simulink model "dialysisDemo"  (R2023a)
settings: Solver=VariableStepAuto  StartTime=0.0  StopTime=3600*4  RelTol=1e-3
libraries: SignalEditorBlockLib x3
settings Model: PacingRate=500  Creator=alibacon  LastModifiedBy=ppatel
settings DebuggingCC: SubsystemReferenceDiagnosticForUnitTest=warning

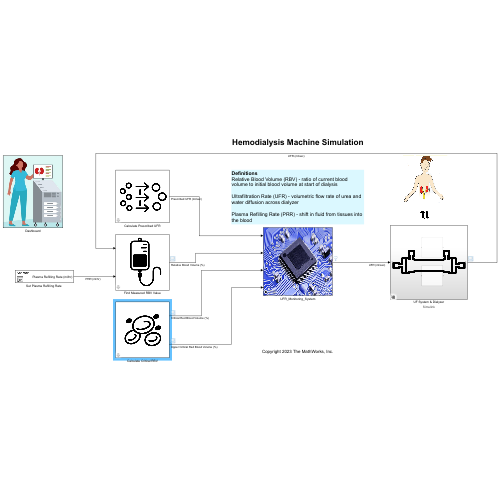
[thumbnail: Simulink's stored preview of the top-level diagram]
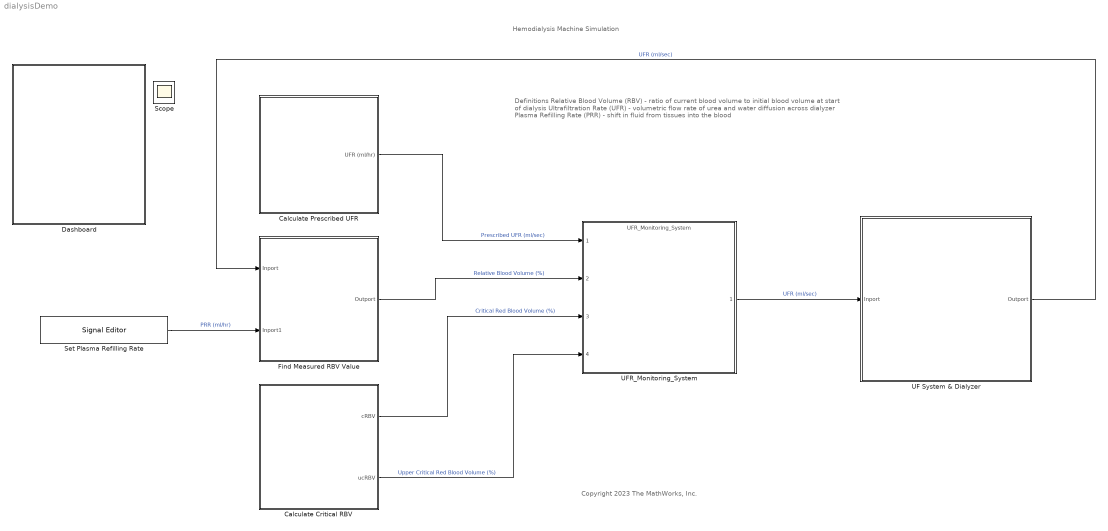
== system dialysisDemo ==
  note: Hemodialysis Machine Simulation
  note: Copyright 2023 The MathWorks, Inc.
  note: Definitions
      | Relative Blood Volume (RBV) - ratio of current blood volume to initial blood volume at start of dialysis
      |
      | Ultrafiltration Rate (UFR) - volumetric flow rate of urea and water diffusion across dialyzer
      |
      | Plasma Refilling Rate (PRR) - shift in fluid from tissues into the blood
  Calculate Critical RBV : Subsystem  mask{BPd=80, UF=2.6, DW=70.6, age=69, arrh=0, chf=0}
      mask prompts: BPd "Diastolic Blood Pressure (mmHg)"; UF "Target Ultrafiltration Volume (L)"; DW "Target Post-Dialysis Dry Weight (kg)"; age "Age (years)"; arrh "Prevalance of Arrythmia"; chf "Prevalance of Congestive Heart Failure Diagnosis"
      mask Display: image('medical-icons-red-blood-cell.png'); % Use "Edit Image" on toolstrip to change.
  Calculate Prescribed UFR : Subsystem  mask{predw=73.2, postdw=70.6, dtime=4}
      mask prompts: predw "Pre-Dialysis Weight (kg)"; postdw "Post-Dialysis Weight (kg)"; dtime "Dialysis Treatment Time (hr)"
      mask Display: image('medical-icons-ufr.png'); % Use "Edit Image" on toolstrip to change.
  Dashboard : Subsystem
      mask Display: image('Dashboard_Input.jpg'); % Use "Edit Image" on toolstrip to change.
  Find Measured RBV Value : Subsystem  mask{BV0=3.774}
      mask prompts: BV0 "Initial Blood Volume (L)"
      mask Display: image('medical-icons-iv-bag.png'); % Use "Edit Image" on toolstrip to change.
  "Set Plasma Refilling Rate " : SignalEditorBlockLib/Signal Editor  FileName=dialysisDemo_PRR.mat  ActiveScenario=Scenario  ActiveSignal=Plasma Refilling Rate (ml/hr)  IsBus=off  OutputBusObjectStr=Bus: BusObject  SampleTime=0  Interpolate=off  ZeroCross=off  OutputAfterFinalValue=Setting to zero  Unit=inherit  PreserveSignalName=on  ApplySigPropsToAllScenarios=on
  UF System & Dialyzer : Subsystem  Variant=on  VariantControlMode=label  VariantControl=Choice  LabelModeActiveChoice=Simulink
      settings: AttributesFormatString=%<LabelModeActiveChoice>
  UFR_Monitoring_System : ModelReference  ModelNameDialog=UFR_Monitoring_System  SimulationMode=Normal  ModelReferenceVersion=3.74
      mask Display: image('Microcontroller.webp'); % Use "Edit Image" on toolstrip to change.
  Scope : Scope
  wires:
  "Set Plasma Refilling Rate "/1 -> Find Measured RBV Value/2(Inport1)  "PRR (ml/hr)"
  UFR_Monitoring_System/1 -> UF System & Dialyzer/1(Inport)  "UFR (ml/sec)"
  UF System & Dialyzer/1(Outport) -> Find Measured RBV Value/1(Inport)  "UFR (ml/sec)"
  Calculate Prescribed UFR/1(UFR (ml/hr)) -> UFR_Monitoring_System/1  "Prescribed UFR (ml/sec)"
  Find Measured RBV Value/1(Outport) -> UFR_Monitoring_System/2  "Relative Blood Volume (%)"
  Calculate Critical RBV/1(cRBV) -> UFR_Monitoring_System/3  "Critical Red Blood Volume (%)"
  Calculate Critical RBV/2(ucRBV) -> UFR_Monitoring_System/4  "Upper Critical Red Blood Volume (%)"

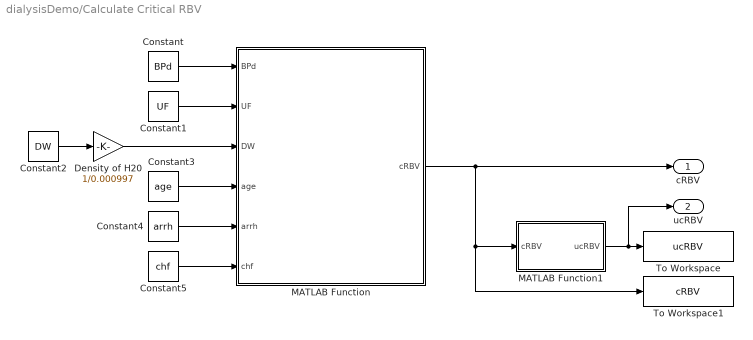
== system dialysisDemo/Calculate Critical RBV ==
  Constant : Constant  Value=BPd
  Constant1 : Constant  Value=UF
  Constant2 : Constant  Value=DW
  Constant3 : Constant  Value=age
  Constant4 : Constant  Value=arrh
  Constant5 : Constant  Value=chf
  Density of H20 : Gain  Gain=1/0.000997
  MATLAB Function : MATLAB Function  TreatAsAtomicUnit=on
  MATLAB Function1 : MATLAB Function  TreatAsAtomicUnit=on
  To Workspace : ToWorkspace  VariableName=ucRBV  SampleTime=-1
  To Workspace1 : ToWorkspace  VariableName=cRBV  SampleTime=-1
  cRBV : Outport
  ucRBV : Outport  Port=2
  wires:
  Constant/1 -> MATLAB Function/1(BPd)
  Constant5/1 -> MATLAB Function/6(chf)
  Constant4/1 -> MATLAB Function/5(arrh)
  Constant3/1 -> MATLAB Function/4(age)
  Constant2/1 -> Density of H20/1
  Constant1/1 -> MATLAB Function/2(UF)
  Density of H20/1 -> MATLAB Function/3(DW)
  MATLAB Function1/1(ucRBV) -> ucRBV/1, To Workspace/1
  MATLAB Function/1(cRBV) -> cRBV/1, To Workspace1/1, MATLAB Function1/1(cRBV)

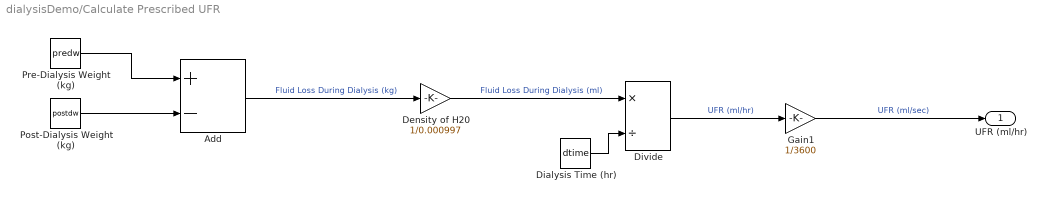
== system dialysisDemo/Calculate Prescribed UFR ==
  Add : Sum  Inputs=+-
  Density of H20 : Gain  Gain=1/0.000997
  Dialysis Time (hr) : Constant  Value=dtime
  Divide : Product  Inputs=*/
  Gain1 : Gain  Gain=1/3600
  Post-Dialysis Weight (kg) : Constant  Value=postdw
  Pre-Dialysis Weight (kg) : Constant  Value=predw
  UFR (ml/hr) : Outport
  wires:
  Add/1 -> Density of H20/1  "Fluid Loss During Dialysis (kg)"
  Divide/1 -> Gain1/1  "UFR (ml/hr)"
  Pre-Dialysis Weight (kg)/1 -> Add/1
  Density of H20/1 -> Divide/1  "Fluid Loss During Dialysis (ml)"
  Post-Dialysis Weight (kg)/1 -> Add/2
  Dialysis Time (hr)/1 -> Divide/2
  Gain1/1 -> UFR (ml/hr)/1  "UFR (ml/sec)"

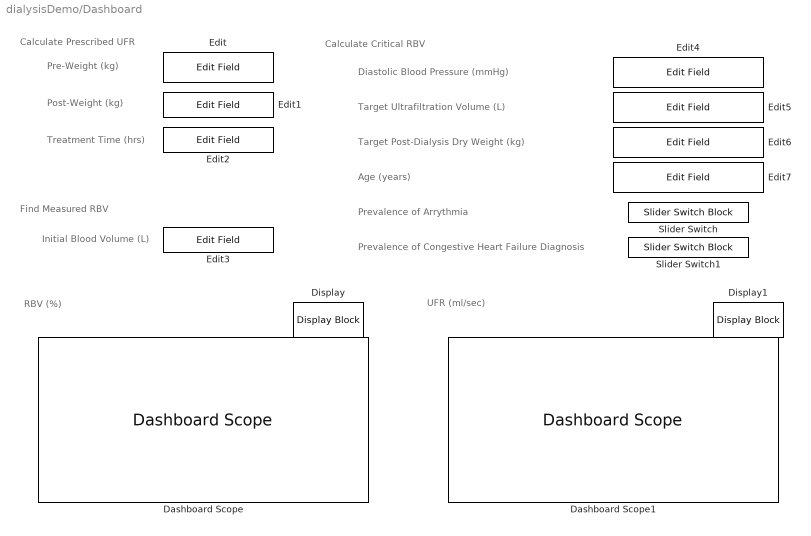
== system dialysisDemo/Dashboard ==
  note: UFR (ml/sec)
  note: RBV (%)
  note: Calculate Critical RBV
  note: Find Measured RBV
  note: Pre-Weight (kg)
  note: Calculate Prescribed UFR
  note: Post-Weight (kg)
  note: Treatment Time (hrs)
  note: Initial Blood Volume (L)
  note: Diastolic Blood Pressure (mmHg)
  note: Target Ultrafiltration Volume (L)
  note: Target Post-Dialysis Dry Weight (kg)
  note: Age (years)
  note: Prevalence of Arrythmia
  note: Prevalence of Congestive Heart Failure Diagnosis
  Dashboard Scope : DashboardScope
  Dashboard Scope1 : DashboardScope
  Display : DisplayBlock  LabelPosition=Hide  Format=Custom  Transparency=1  Layout=Fill available space  FormatString=%.2f
  Display1 : DisplayBlock  LabelPosition=Hide  Format=Custom  Transparency=1  FormatString=%.2f
  Edit{,1..7} (8 alike) : EditField  LabelPosition=Hide  ShowInitialText=on  Alignment=Center
  Slider Switch : SliderSwitchBlock  LabelPosition=Hide
      settings: Values={{'No', 'Yes'}, [0 1]}
  Slider Switch1 : SliderSwitchBlock  LabelPosition=Hide
      settings: Values={{'No', 'Yes'}, [0 1]}

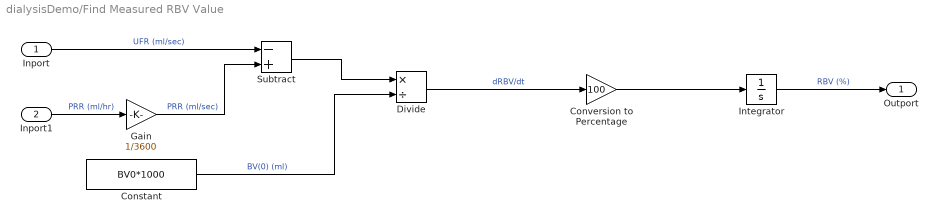
== system dialysisDemo/Find Measured RBV Value ==
  Inport : Inport
  Inport1 : Inport  Port=2
  Constant : Constant  Value=BV0*1000
  Conversion to Percentage : Gain  Gain=100
  Divide : Product  Inputs=*/
  Gain : Gain  Gain=1/3600
  Integrator : Integrator  InitialCondition=100
  Subtract : Sum  Inputs=-+
  Outport : Outport
  wires:
  Integrator/1 -> Outport/1  "RBV (%)"
  Divide/1 -> Conversion to Percentage/1  "dRBV/dt"
  Subtract/1 -> Divide/1
  Constant/1 -> Divide/2  "BV(0) (ml)"
  Inport/1 -> Subtract/1  "UFR (ml/sec)"
  Inport1/1 -> Gain/1  "PRR (ml/hr)"
  Conversion to Percentage/1 -> Integrator/1
  Gain/1 -> Subtract/2  "PRR (ml/sec)"

== system dialysisDemo/UF System & Dialyzer ==
  Inport : Inport
  Simscape Model : Subsystem  VariantControl=Simscape  ReferencedSubsystem=Simscape_UF_Model  DFR=30000
  Simulink Model : Subsystem  VariantControl=Simulink  mask{DFR=30000}
      mask prompts: DFR "Dialysate Pump Flow Rate (ml/hr)"
      mask Display: image('medical-icons-dialyzer.png'); % Use "Edit Image" on toolstrip to change.
  Outport : Outport

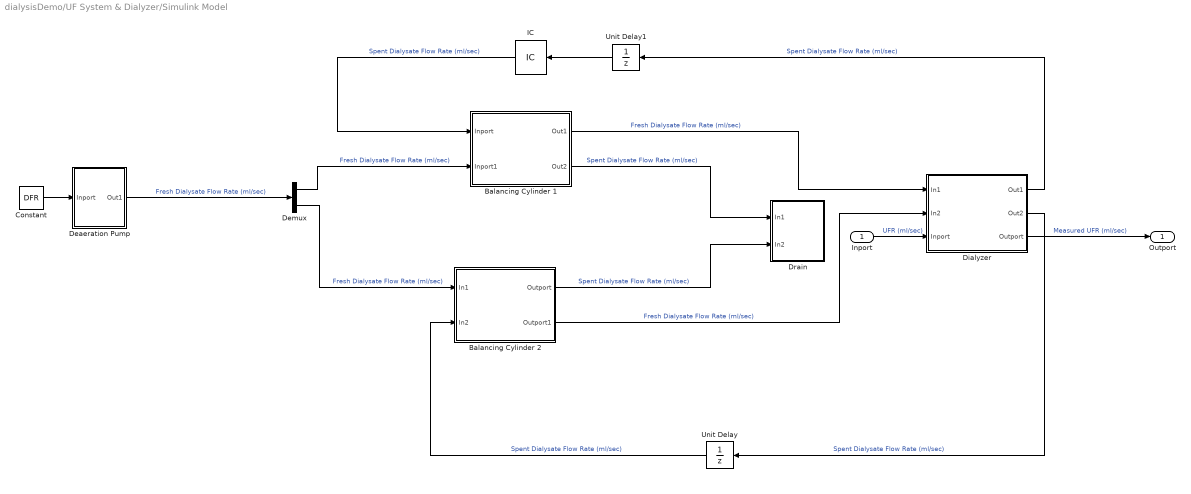
== system dialysisDemo/UF System & Dialyzer/Simulink Model ==
  Inport : Inport
  Balancing Cylinder 1 : Subsystem
  Balancing Cylinder 2 : Subsystem
  Constant : Constant  Value=DFR
  Deaeration Pump : Subsystem
  Demux : Demux  Outputs=2
  Dialyzer : Subsystem
  Drain : Subsystem
  IC : InitialCondition  Value=DFR
  Unit Delay : UnitDelay  SampleTime=-1  HasFrameUpgradeWarning=on
  Unit Delay1 : UnitDelay  SampleTime=-1  HasFrameUpgradeWarning=on
  Outport : Outport
  wires:
  Dialyzer/3(Outport) -> Outport/1  "Measured UFR (ml/sec)"
  Inport/1 -> Dialyzer/3(Inport)  "UFR (ml/sec)"
  Dialyzer/2(Out2) -> Unit Delay/1  "Spent Dialysate Flow Rate (ml/sec)"
  Constant/1 -> Deaeration Pump/1(Inport)
  Balancing Cylinder 1/2(Out2) -> Drain/1(In1)  "Spent Dialysate Flow Rate (ml/sec)"
  Demux/1 -> Balancing Cylinder 1/2(Inport1)  "Fresh Dialysate Flow Rate (ml/sec)"
  Balancing Cylinder 2/1(Outport) -> Drain/2(In2)  "Spent Dialysate Flow Rate (ml/sec)"
  Balancing Cylinder 1/1(Out1) -> Dialyzer/1(In1)  "Fresh Dialysate Flow Rate (ml/sec)"
  Unit Delay/1 -> Balancing Cylinder 2/2(In2)  "Spent Dialysate Flow Rate (ml/sec)"
  Unit Delay1/1 -> IC/1
  Demux/2 -> Balancing Cylinder 2/1(In1)  "Fresh Dialysate Flow Rate (ml/sec)"
  Dialyzer/1(Out1) -> Unit Delay1/1  "Spent Dialysate Flow Rate (ml/sec)"
  Deaeration Pump/1(Out1) -> Demux/1  "Fresh Dialysate Flow Rate (ml/sec)"
  Balancing Cylinder 2/2(Outport1) -> Dialyzer/2(In2)  "Fresh Dialysate Flow Rate (ml/sec)"
  IC/1 -> Balancing Cylinder 1/1(Inport)  "Spent Dialysate Flow Rate (ml/sec)"

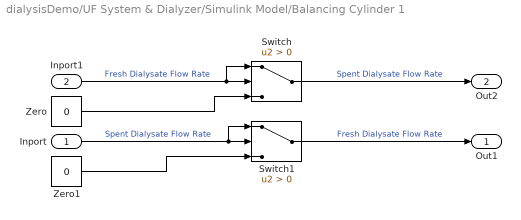
== system dialysisDemo/UF System & Dialyzer/Simulink Model/Balancing Cylinder 1 ==
  Inport : Inport
  Inport1 : Inport  Port=2
  Switch : Switch  Criteria=u2 > Threshold  SaturateOnIntegerOverflow=off  InputSameDT=off
  Switch1 : Switch  Criteria=u2 > Threshold  SaturateOnIntegerOverflow=off  InputSameDT=off
  Zero : Constant  Value=0  OutDataTypeStr=Inherit: Inherit via back propagation
  Zero1 : Constant  Value=0  OutDataTypeStr=Inherit: Inherit via back propagation
  Out1 : Outport
  Out2 : Outport  Port=2
  wires:
  Zero1/1 -> Switch1/3
  Zero/1 -> Switch/3
  Switch/1 -> Out2/1  "Spent Dialysate Flow Rate"
  Switch1/1 -> Out1/1  "Fresh Dialysate Flow Rate"
  Inport/1 -> Switch1/2, Switch1/1  "Spent Dialysate Flow Rate"
  Inport1/1 -> Switch/2, Switch/1  "Fresh Dialysate Flow Rate"

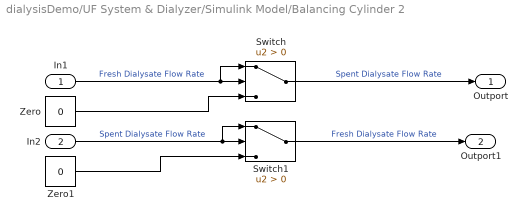
== system dialysisDemo/UF System & Dialyzer/Simulink Model/Balancing Cylinder 2 ==
  In1 : Inport
  In2 : Inport  Port=2
  Switch : Switch  Criteria=u2 > Threshold  SaturateOnIntegerOverflow=off  InputSameDT=off
  Switch1 : Switch  Criteria=u2 > Threshold  SaturateOnIntegerOverflow=off  InputSameDT=off
  Zero : Constant  Value=0  OutDataTypeStr=Inherit: Inherit via back propagation
  Zero1 : Constant  Value=0  OutDataTypeStr=Inherit: Inherit via back propagation
  Outport : Outport
  Outport1 : Outport  Port=2
  wires:
  Zero1/1 -> Switch1/3
  Zero/1 -> Switch/3
  Switch/1 -> Outport/1  "Spent Dialysate Flow Rate"
  Switch1/1 -> Outport1/1  "Fresh Dialysate Flow Rate"
  In2/1 -> Switch1/2, Switch1/1  "Spent Dialysate Flow Rate"
  In1/1 -> Switch/2, Switch/1  "Fresh Dialysate Flow Rate"

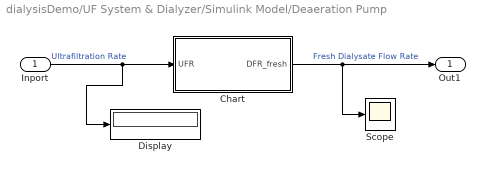
== system dialysisDemo/UF System & Dialyzer/Simulink Model/Deaeration Pump ==
  Inport : Inport
  Chart : Stateflow chart  TreatAsAtomicUnit=on
  Display : Display
  Scope : Scope
  Out1 : Outport
  wires:
  Chart/1(DFR_fresh) -> Out1/1, Scope/1  "Fresh Dialysate Flow Rate"
  Inport/1 -> Chart/1(UFR), Display/1  "Ultrafiltration Rate"

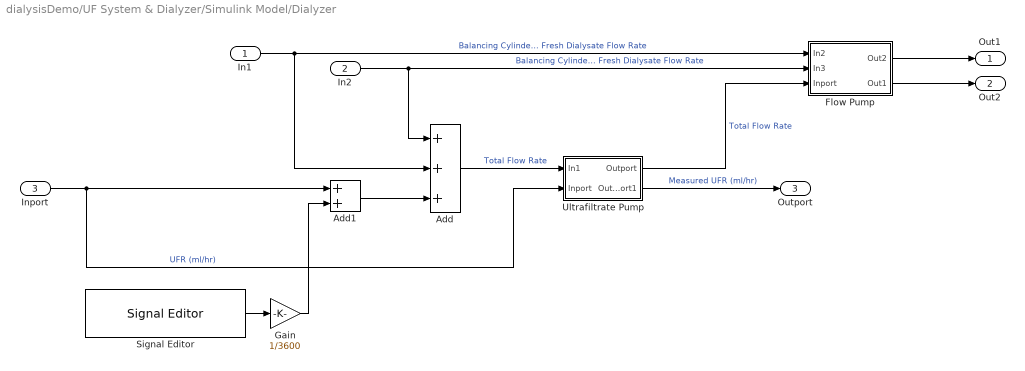
== system dialysisDemo/UF System & Dialyzer/Simulink Model/Dialyzer ==
  In1 : Inport
  In2 : Inport  Port=2
  Inport : Inport  Port=3
  Add : Sum  Inputs=+++
  Add1 : Sum
  Flow Pump : Subsystem
  Gain : Gain  Gain=1/3600
  Signal Editor : SignalEditorBlockLib/Signal Editor  FileName=dialysisDemo_noise.mat  ActiveScenario=UltrafiltrationRate  ActiveSignal=UFR Noise (ml/hr)  IsBus=off  OutputBusObjectStr=Bus: BusObject  SampleTime=0  Interpolate=off  ZeroCross=off  OutputAfterFinalValue=Setting to zero  Unit=inherit  PreserveSignalName=on  ApplySigPropsToAllScenarios=on
  Ultrafiltrate Pump : Subsystem
  Out1 : Outport
  Out2 : Outport  Port=2
  Outport : Outport  Port=3
  wires:
  Gain/1 -> Add1/2
  Signal Editor/1 -> Gain/1
  Add1/1 -> Add/3
  Ultrafiltrate Pump/2(Outport1) -> Outport/1  "Measured UFR (ml/hr)"
  Inport/1 -> Ultrafiltrate Pump/2(Inport), Add1/1  "UFR (ml/hr)"
  Ultrafiltrate Pump/1(Outport) -> Flow Pump/3(Inport)  "Total Flow Rate"
  Flow Pump/1(Out2) -> Out1/1
  Flow Pump/2(Out1) -> Out2/1
  Add/1 -> Ultrafiltrate Pump/1(In1)  "Total Flow Rate"
  In1/1 -> Flow Pump/1(In2), Add/2  "Balancing Cylinder 1 Fresh Dialysate Flow Rate"
  In2/1 -> Flow Pump/2(In3), Add/1  "Balancing Cylinder 2 Fresh Dialysate Flow Rate"

== system dialysisDemo/UF System & Dialyzer/Simulink Model/Drain ==
  In1 : Inport
  In2 : Inport  Port=2
  Terminator : Terminator
  Terminator1 : Terminator
  wires:
  In2/1 -> Terminator1/1
  In1/1 -> Terminator/1

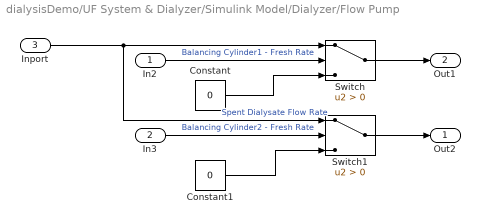
== system dialysisDemo/UF System & Dialyzer/Simulink Model/Dialyzer/Flow Pump ==
  In2 : Inport
  In3 : Inport  Port=2
  Inport : Inport  Port=3
  Constant : Constant  Value=0  SampleTime=-1
  Constant1 : Constant  Value=0  SampleTime=-1
  Switch : Switch  Criteria=u2 > Threshold  SaturateOnIntegerOverflow=off  InputSameDT=off
  Switch1 : Switch  Criteria=u2 > Threshold  SaturateOnIntegerOverflow=off  InputSameDT=off
  Out2 : Outport
  Out1 : Outport  Port=2
  wires:
  Constant1/1 -> Switch1/3
  Switch1/1 -> Out2/1
  In3/1 -> Switch1/2  "Balancing Cylinder2 - Fresh Rate"
  Constant/1 -> Switch/3
  Switch/1 -> Out1/1
  In2/1 -> Switch/2  "Balancing Cylinder1 - Fresh Rate"
  Inport/1 -> Switch1/1, Switch/1  "Spent Dialysate Flow Rate"

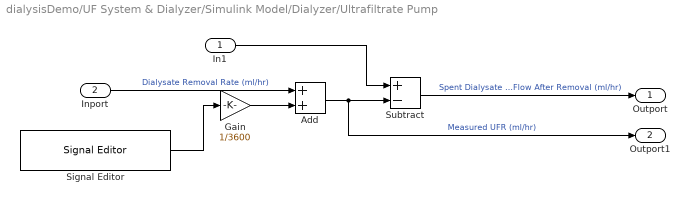
== system dialysisDemo/UF System & Dialyzer/Simulink Model/Dialyzer/Ultrafiltrate Pump ==
  In1 : Inport
  Inport : Inport  Port=2
  Add : Sum
  Gain : Gain  Gain=1/3600
  Signal Editor : SignalEditorBlockLib/Signal Editor  FileName=dialysisDemo_noise.mat  ActiveScenario=UltrafiltratePump  ActiveSignal=UF Pump Noise (ml/hr)  IsBus=off  OutputBusObjectStr=Bus: BusObject  SampleTime=0  Interpolate=off  ZeroCross=off  OutputAfterFinalValue=Setting to zero  Unit=inherit  PreserveSignalName=on  ApplySigPropsToAllScenarios=on
  Subtract : Sum  Inputs=+-
  Outport : Outport
  Outport1 : Outport  Port=2
  wires:
  Gain/1 -> Add/2
  Signal Editor/1 -> Gain/1
  Add/1 -> Subtract/2, Outport1/1  "Measured UFR (ml/hr)"
  Inport/1 -> Add/1  "Dialysate Removal Rate (ml/hr)"
  Subtract/1 -> Outport/1  "Spent Dialysate Flow After Removal (ml/hr)"
  In1/1 -> Subtract/1

== matlab function dialysisDemo/Calculate Critical RBV/MATLAB Function ==
  data: BPd input; cRBV output; UF input; DW input; age input; arrh input; chf input
function cRBV = calculate_cRBV(BPd, UF, DW, age, arrh, chf)
% BPd - diastolic blood pressure at t=0 (mmHg)
% UF -  (l)
% DW - target dry weight post-dialysis (l)
% age - age in years (yrs)
% arrh - prevalence of arrythmia (0=absent; 1=existent)
% chf - prevalence of congestive heart failure diagnosis (0=absent; 1=existent)

cRBV = 97.8 - 0.08*BPd - (UF/DW) + 0.05*age + 1.5*arrh + 0.2*chf;

== stateflow chart dialysisDemo/UF System & Dialyzer/Simulink Model/Deaeration Pump/Chart ==
  state FillCylinder2
    entry: DFR_fresh = [UFR, 0];
    during: DFR_fresh = [UFR, 0];
  state FillCylinder1
    entry: DFR_fresh = [0, UFR];
    during: DFR_fresh = [0, UFR];
  (default) -> FillCylinder1
  FillCylinder2 -> FillCylinder1 : after(30*3600/UFR, sec)
  FillCylinder1 -> FillCylinder2 : after(30*3600/UFR, sec)
  data: UFR input; DFR_fresh output

== matlab function dialysisDemo/Calculate Critical RBV/MATLAB Function1 ==
  data: cRBV input; ucRBV output
function ucRBV = fcn(cRBV)
% Calculate the upper threshold for cRBV where UFR begins to decrease
ucRBV = (100 - cRBV) / 2 + cRBV;
